simulink model "modelo_completo_sim"  (R2022b)
settings: Solver=VariableStepAuto  StartTime=0.0  StopTime=10.0  RelTol=1e-3
values from neighbouring files (symbols this model uses):
  alpha_Cu = 3.9e-3    (= 0.0039)    [analisis_estabilidad.m]    (also in parametros.m; parametros_sim.m)
  b_eq = b_eq_max    (= 2.40277777778e-05)    [analisis_estabilidad.m]    (also in parametros.m = 2.19444444444e-05; parametros_sim.m = 2.19444444444e-05)
  C_ts = 0.818    [analisis_estabilidad.m]    (also in parametros.m; parametros_sim.m)
  g = 9.80665    [analisis_estabilidad.m]    (also in parametros.m; parametros_sim.m)
  J_eq = J_eq_max    (= 4.58263888889e-05)    [analisis_estabilidad.m]    (also in parametros.m = 1.97847222222e-05; parametros_sim.m = 1.97847222222e-05)
  k_l = (m*l_cm + m_l*l_l)*g    (= 2.4516625)    [analisis_estabilidad.m]    (also in parametros.m = 0.25; parametros_sim.m)
  L_d = 6.6    [analisis_estabilidad.m]    (also in parametros.m = 0.0066; parametros_sim.m; polosyceros.m = L_d^3)
  L_ls = 0.8    [analisis_estabilidad.m]    (also in parametros.m = 0.0008; parametros_sim.m)
  L_q = 5.8    [analisis_estabilidad.m]    (also in parametros.m = 0.0058; parametros_sim.m; polosyceros.m = L_q^3)
  lambda_m = 0.016    [analisis_estabilidad.m]    (also in parametros.m; parametros_sim.m)
  P_p = 3    [analisis_estabilidad.m]    (also in parametros.m; parametros_sim.m)
  r = 120    [analisis_estabilidad.m]    (also in parametros.m; parametros_sim.m)
  R_s_ref = 1.02    [analisis_estabilidad.m]    (also in parametros.m; parametros_sim.m)
  R_ts_amb = 146.7    [analisis_estabilidad.m]    (also in parametros.m; parametros_sim.m)
  T_s_ref = 20    [analisis_estabilidad.m]    (also in parametros.m; parametros_sim.m)
settings Model: Creator=martinarobyculasso  LastModifiedBy=martinarobyculasso

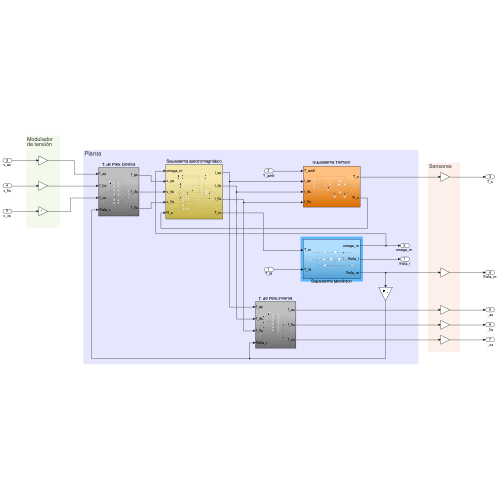
[thumbnail: Simulink's stored preview of the top-level diagram]
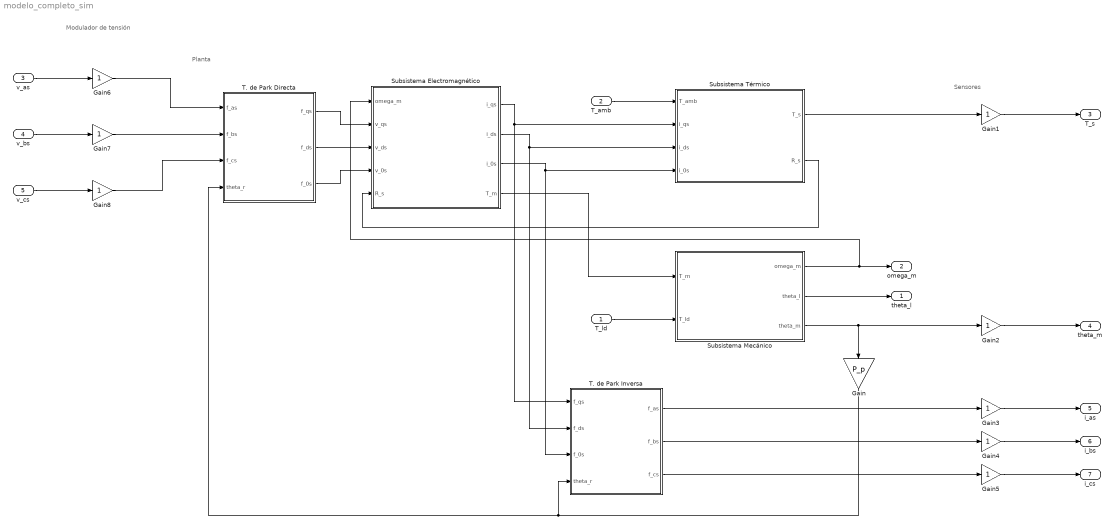
== system modelo_completo_sim ==
  note: Sensores
  note: Modulador
      | de tensión
  note: Planta
  T_ld : Inport
  T_amb : Inport  Port=2
  v_as : Inport  Port=3
  v_bs : Inport  Port=4
  v_cs : Inport  Port=5
  Gain : Gain  Gain=P_p
  Gain{1..8} (8 alike) : Gain
  Subsistema Electromagnético : Subsystem
  Subsistema Mecánico : Subsystem
  Subsistema Térmico : Subsystem
  T. de Park Directa : Subsystem
  T. de Park Inversa : Subsystem
  theta_l : Outport
  "omega_m " : Outport  Port=2
  T_s : Outport  Port=3
  theta_m : Outport  Port=4
  i_as : Outport  Port=5
  i_bs : Outport  Port=6
  i_cs : Outport  Port=7
  wires:
  T. de Park Directa/1(f_qs) -> Subsistema Electromagnético/2(v_qs)
  T. de Park Directa/2(f_ds) -> Subsistema Electromagnético/3(v_ds)
  T. de Park Directa/3(f_0s) -> Subsistema Electromagnético/4(v_0s)
  Subsistema Electromagnético/1(i_qs) -> T. de Park Inversa/1(f_qs), Subsistema Térmico/2(i_qs)
  Subsistema Electromagnético/2(i_ds) -> T. de Park Inversa/2(f_ds), Subsistema Térmico/3(i_ds)
  Subsistema Electromagnético/3(i_0s) -> T. de Park Inversa/3(f_0s), Subsistema Térmico/4(i_0s)
  Subsistema Térmico/2(R_s) -> Subsistema Electromagnético/5(R_s)
  Subsistema Electromagnético/4(T_m) -> Subsistema Mecánico/1(T_m)
  Subsistema Mecánico/1(omega_m) -> "omega_m "/1, Subsistema Electromagnético/1(omega_m)
  T_ld/1 -> Subsistema Mecánico/2(T_ld)
  T_amb/1 -> Subsistema Térmico/1(T_amb)
  Subsistema Mecánico/2(theta_l) -> theta_l/1
  Subsistema Mecánico/3(theta_m) -> Gain/1, Gain2/1
  Gain/1 -> T. de Park Directa/4(theta_r), T. de Park Inversa/4(theta_r)
  Subsistema Térmico/1(T_s) -> Gain1/1
  T. de Park Inversa/1(f_as) -> Gain3/1
  T. de Park Inversa/2(f_bs) -> Gain4/1
  T. de Park Inversa/3(f_cs) -> Gain5/1
  Gain7/1 -> T. de Park Directa/2(f_bs)
  Gain6/1 -> T. de Park Directa/1(f_as)
  Gain8/1 -> T. de Park Directa/3(f_cs)
  v_cs/1 -> Gain8/1
  v_bs/1 -> Gain7/1
  v_as/1 -> Gain6/1
  Gain5/1 -> i_cs/1
  Gain4/1 -> i_bs/1
  Gain3/1 -> i_as/1
  Gain2/1 -> theta_m/1
  Gain1/1 -> T_s/1

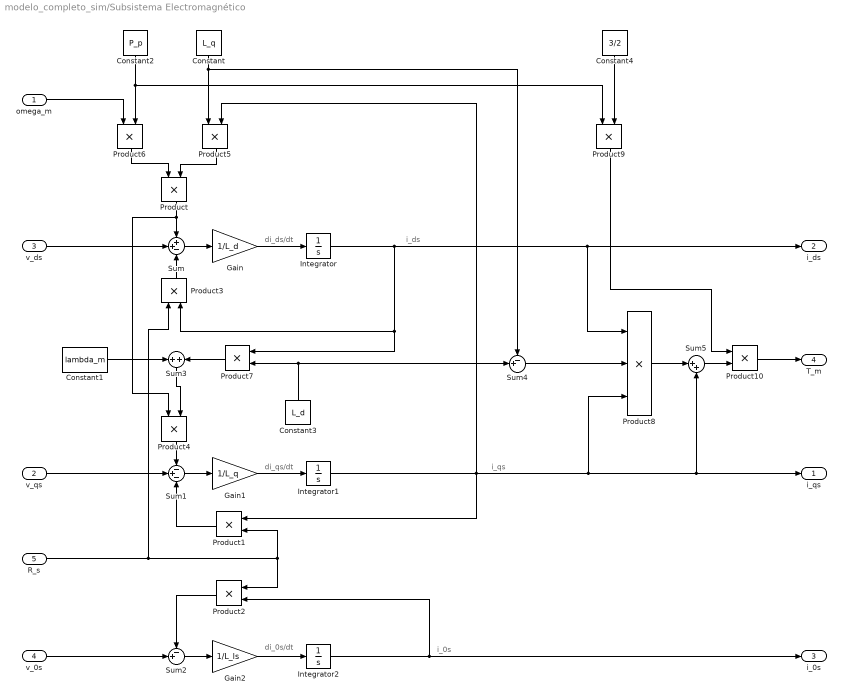
== system modelo_completo_sim/Subsistema Electromagnético ==
  note: i_0s
  note: di_0s/dt
  note: i_qs
  note: i_ds
  note: di_ds/dt
  note: di_qs/dt
  omega_m : Inport
  v_qs : Inport  Port=2
  v_ds : Inport  Port=3
  v_0s : Inport  Port=4
  R_s : Inport  Port=5
  Constant : Constant  Value=L_q
  Constant1 : Constant  Value=lambda_m
  Constant2 : Constant  Value=P_p
  Constant3 : Constant  Value=L_d
  Constant4 : Constant  Value=3/2
  Gain : Gain  Gain=1/L_d
  Gain1 : Gain  Gain=1/L_q
  Gain2 : Gain  Gain=1/L_ls
  Integrator : Integrator
  Integrator1 : Integrator
  Integrator2 : Integrator
  Product{,1..7,9..10} (10 alike) : Product
  Product8 : Product  Inputs=3
  Sum : Sum  Inputs=++-
  Sum1 : Sum  Inputs=-+-
  Sum2 : Sum  Inputs=-+|
  Sum3 : Sum  Inputs=+|+
  Sum4 : Sum  Inputs=-+|
  Sum5 : Sum  Inputs=|++
  i_qs : Outport
  i_ds : Outport  Port=2
  i_0s : Outport  Port=3
  T_m : Outport  Port=4
  wires:
  Product4/1 -> Sum1/1
  Product1/1 -> Sum1/3
  Sum2/1 -> Gain2/1
  Product/1 -> Product4/1, Sum/1
  v_0s/1 -> Sum2/2
  v_qs/1 -> Sum1/2
  Gain2/1 -> Integrator2/1
  Product2/1 -> Sum2/1
  Integrator2/1 -> i_0s/1, Product2/2
  Integrator/1 -> Product8/1, i_ds/1, Product7/1, Product3/2
  Sum3/1 -> Product4/2
  Sum/1 -> Gain/1
  R_s/1 -> Product3/1, Product2/1, Product1/2
  Gain1/1 -> Integrator1/1
  Gain/1 -> Integrator/1
  Constant1/1 -> Sum3/1
  Product3/1 -> Sum/3
  Integrator1/1 -> Product8/3, i_qs/1, Sum5/2, Product5/2, Product1/1
  Sum1/1 -> Gain1/1
  v_ds/1 -> Sum/2
  Constant/1 -> Sum4/1, Product5/1
  Product5/1 -> Product/2
  Constant2/1 -> Product9/1, Product6/2
  omega_m/1 -> Product6/1
  Product6/1 -> Product/1
  Product7/1 -> Sum3/2
  Constant3/1 -> Product7/2, Sum4/2
  Sum4/1 -> Product8/2
  Product8/1 -> Sum5/1
  Constant4/1 -> Product9/2
  Sum5/1 -> Product10/2
  Product9/1 -> Product10/1
  Product10/1 -> T_m/1

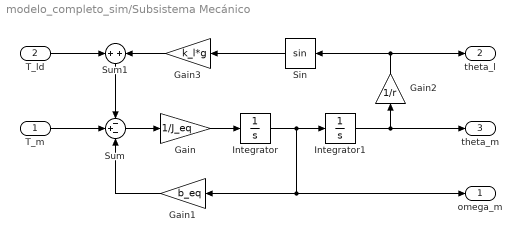
== system modelo_completo_sim/Subsistema Mecánico ==
  T_m : Inport
  T_ld : Inport  Port=2
  Gain : Gain  Gain=1/J_eq
  Gain1 : Gain  Gain=b_eq
  Gain2 : Gain  Gain=1/r
  Gain3 : Gain  Gain=k_l*g
  Integrator : Integrator
  Integrator1 : Integrator
  Sin : Trigonometry
  Sum : Sum  Inputs=-+-
  Sum1 : Sum
  omega_m : Outport
  theta_l : Outport  Port=2
  theta_m : Outport  Port=3
  wires:
  T_m/1 -> Sum/2
  Sin/1 -> Gain3/1
  T_ld/1 -> Sum1/1
  Gain2/1 -> theta_l/1, Sin/1
  Gain1/1 -> Sum/3
  Gain3/1 -> Sum1/2
  Integrator1/1 -> theta_m/1, Gain2/1
  Sum/1 -> Gain/1
  Gain/1 -> Integrator/1
  Sum1/1 -> Sum/1
  Integrator/1 -> Integrator1/1, omega_m/1, Gain1/1

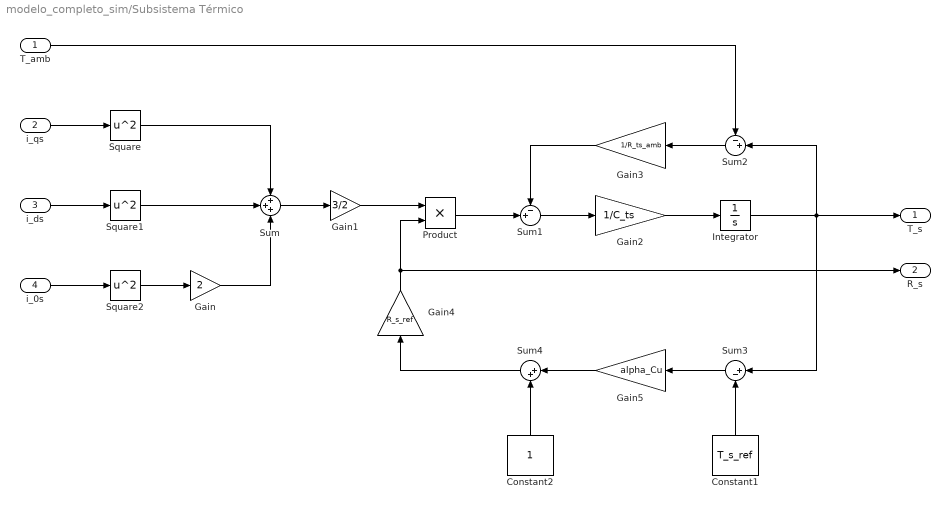
== system modelo_completo_sim/Subsistema Térmico ==
  T_amb : Inport
  i_qs : Inport  Port=2
  i_ds : Inport  Port=3
  i_0s : Inport  Port=4
  Constant1 : Constant  Value=T_s_ref
  Constant2 : Constant
  Gain : Gain  Gain=2
  Gain1 : Gain  Gain=3/2
  Gain2 : Gain  Gain=1/C_ts
  Gain3 : Gain  Gain=1/R_ts_amb
  Gain4 : Gain  Gain=R_s_ref
  Gain5 : Gain  Gain=alpha_Cu
  Integrator : Integrator
  Product : Product
  Square : Math  Operator=square
  Square1 : Math  Operator=square
  Square2 : Math  Operator=square
  Sum : Sum  Inputs=+++
  Sum1 : Sum  Inputs=-+|
  Sum2 : Sum  Inputs=-+|
  Sum3 : Sum  Inputs=|+-
  Sum4 : Sum  Inputs=|++
  T_s : Outport
  R_s : Outport  Port=2
  wires:
  Product/1 -> Sum1/2
  Gain1/1 -> Product/1
  Sum4/1 -> Gain4/1
  Sum3/1 -> Gain5/1
  Constant1/1 -> Sum3/2
  Sum2/1 -> Gain3/1
  Gain3/1 -> Sum1/1
  Sum1/1 -> Gain2/1
  i_ds/1 -> Square1/1
  Gain4/1 -> R_s/1, Product/2
  Gain2/1 -> Integrator/1
  Sum/1 -> Gain1/1
  Gain/1 -> Sum/3
  Square/1 -> Sum/1
  Square1/1 -> Sum/2
  Integrator/1 -> T_s/1, Sum3/1, Sum2/2
  Gain5/1 -> Sum4/1
  Square2/1 -> Gain/1
  i_0s/1 -> Square2/1
  Constant2/1 -> Sum4/2
  i_qs/1 -> Square/1
  T_amb/1 -> Sum2/1

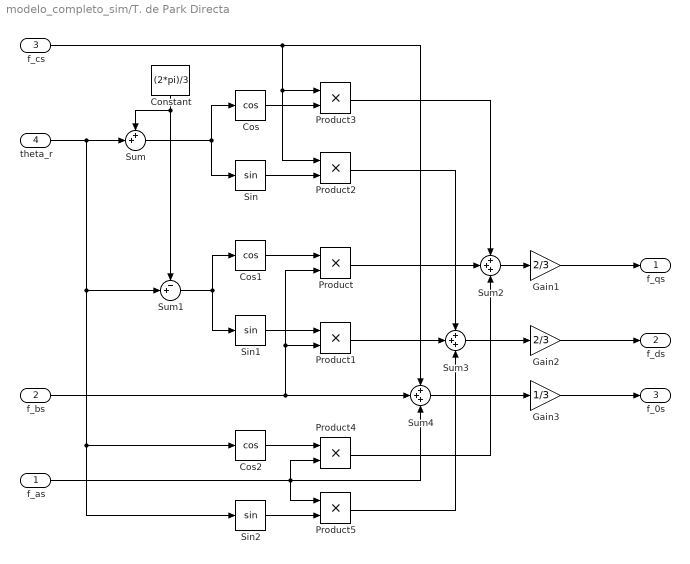
== system modelo_completo_sim/T. de Park Directa ==
  f_as : Inport
  f_bs : Inport  Port=2
  f_cs : Inport  Port=3
  theta_r : Inport  Port=4
  Constant : Constant  Value=(2*pi)/3
  Cos : Trigonometry  Operator=cos
  Cos1 : Trigonometry  Operator=cos
  Cos2 : Trigonometry  Operator=cos
  Gain1 : Gain  Gain=2/3
  Gain2 : Gain  Gain=2/3
  Gain3 : Gain  Gain=1/3
  Product{,1..5} (6 alike) : Product
  Sin : Trigonometry
  Sin1 : Trigonometry
  Sin2 : Trigonometry
  Sum : Sum  Inputs=++|
  Sum1 : Sum  Inputs=-+|
  Sum2 : Sum  Inputs=+++
  Sum3 : Sum  Inputs=+++
  Sum4 : Sum  Inputs=+++
  f_qs : Outport
  f_ds : Outport  Port=2
  f_0s : Outport  Port=3
  wires:
  Product4/1 -> Sum2/3
  Cos1/1 -> Product/1
  theta_r/1 -> Sum/2, Sin2/1, Cos2/1, Sum1/2
  Sin1/1 -> Product1/1
  Sin2/1 -> Product5/2
  Product3/1 -> Sum2/1
  Cos2/1 -> Product4/1
  Product1/1 -> Sum3/2
  f_as/1 -> Sum4/3, Product4/2, Product5/1
  Sum2/1 -> Gain1/1
  Sum1/1 -> Sin1/1, Cos1/1
  f_bs/1 -> Sum4/2, Product/2, Product1/2
  Sum/1 -> Sin/1, Cos/1
  Product2/1 -> Sum3/1
  Sin/1 -> Product2/2
  Sum4/1 -> Gain3/1
  Gain1/1 -> f_qs/1
  f_cs/1 -> Sum4/1, Product2/1, Product3/1
  Gain2/1 -> f_ds/1
  Product/1 -> Sum2/2
  Sum3/1 -> Gain2/1
  Cos/1 -> Product3/2
  Constant/1 -> Sum1/1, Sum/1
  Gain3/1 -> f_0s/1
  Product5/1 -> Sum3/3

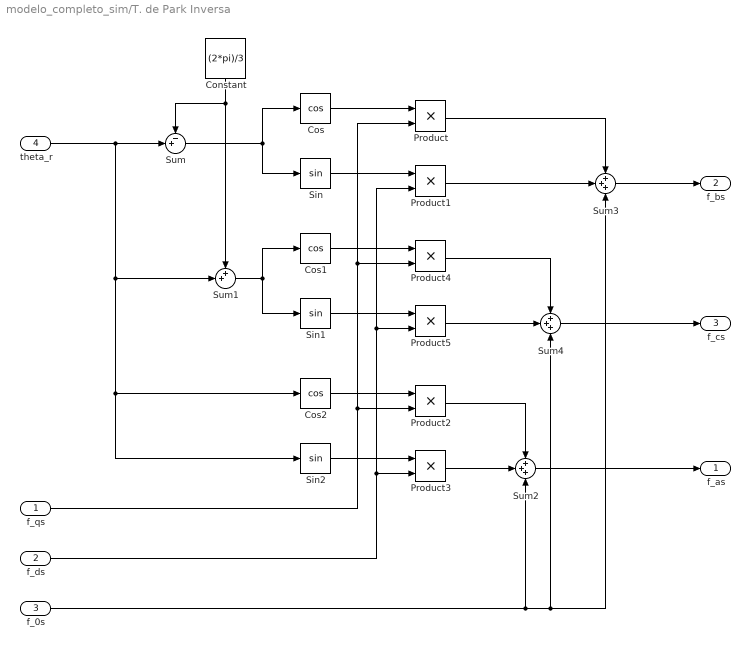
== system modelo_completo_sim/T. de Park Inversa ==
  f_qs : Inport
  f_ds : Inport  Port=2
  f_0s : Inport  Port=3
  theta_r : Inport  Port=4
  Constant : Constant  Value=(2*pi)/3
  Cos : Trigonometry  Operator=cos
  Cos1 : Trigonometry  Operator=cos
  Cos2 : Trigonometry  Operator=cos
  Product{,1..5} (6 alike) : Product
  Sin : Trigonometry
  Sin1 : Trigonometry
  Sin2 : Trigonometry
  Sum : Sum  Inputs=-+|
  Sum1 : Sum  Inputs=++|
  Sum2 : Sum  Inputs=+++
  Sum3 : Sum  Inputs=+++
  Sum4 : Sum  Inputs=+++
  f_as : Outport
  f_bs : Outport  Port=2
  f_cs : Outport  Port=3
  wires:
  Product4/1 -> Sum4/1
  Sum2/1 -> f_as/1
  f_qs/1 -> Product4/2, Product/2, Product2/2
  Sum/1 -> Sin/1, Cos/1
  theta_r/1 -> Sum1/2, Cos2/1, Sin2/1, Sum/2
  Product1/1 -> Sum3/2
  Product3/1 -> Sum2/2
  Product5/1 -> Sum4/2
  Sin1/1 -> Product5/1
  Product/1 -> Sum3/1
  Cos/1 -> Product/1
  Sin2/1 -> Product3/1
  Cos1/1 -> Product4/1
  Sin/1 -> Product1/1
  f_0s/1 -> Sum3/3, Sum4/3, Sum2/3
  Sum3/1 -> f_bs/1
  Sum1/1 -> Sin1/1, Cos1/1
  Cos2/1 -> Product2/1
  Product2/1 -> Sum2/1
  Sum4/1 -> f_cs/1
  f_ds/1 -> Product3/2, Product5/2, Product1/2
  Constant/1 -> Sum/1, Sum1/1
